simulink library "vmc"  (R2021b)
settings: Solver=VariableStepAuto  StartTime=0.0  StopTime=10.0  RelTol=1e-3
undefined symbols (not defined in the file): AVMC_ACCDeltaTqGradeGn_X_deg, AVMC_ACCDeltaTqIGain4OVRD_X_kph, AVMC_ACCDeltaTqIGain4OVRD_Y_mps2, AVMC_ACCDeltaTqIGain_X_kph, AVMC_ACCDeltaTqIGain_Y_mps2, AVMC_ACCDeltaTqPGain_X_kph, AVMC_ACCDeltaTqPGain_Y_kph, AVMC_ACCGradeofst_X_G, AVMC_ACCGradeofst_Y_pct, AVMC_ACCLoSpdTqLoLim4JP_X_kph, AVMC_ACCLoSpdTqLoLim4JP_Y_deg, AVMC_ACCLoSpdTqLowerLim_X_kph, AVMC_ACCLoSpdTqLowerLim_Y_deg, AVMC_ACCReqAccelGain_X_mps2, AVMC_ACCReqAccelGain_Y_enum, AVMC_ADSPosGFBDeltaTq_X_kph, AVMC_ADSPosGFBDeltaTq_Y_mps2, AVMC_AggressJerkPCT4AT_X_kph, AVMC_AggressJerkPCT_X_kph, AVMC_AggressLimitPCT4AT_X_kph, AVMC_AggressLimitPCT_X_kph, AVMC_DECGradeofst_X_G, AVMC_DECGradeofst_Y_pct, AVMC_DISCDeltaTqIGain_X_kph, AVMC_DISCDeltaTqIGain_Y_mps2, AVMC_DISCDeltaTqPGain_X_kph, AVMC_DISCDeltaTqPGain_Y_kph, AVMC_EPSForceSelect_X_enum, AVMC_EPSForceSelect_Y_enum, AVMC_EPSForceSelectD21_X_enum, AVMC_EPSForceSelectD21_Y_enum, AVMC_ESCRegenOut_X_kph, AVMC_ESCRegenOut_Y_Deg, AVMC_ESCRegenOutEnSpd_X_Deg, AVMC_EstPitchSlopeTs_X_kph, AVMC_GradeCompFlt_X_kph, AVMC_GyroYBandLo_X_Gps, AVMC_HoldResTq_X_kph, AVMC_ISOAccLimit_X_mps, AVMC_ISODecLimit_X_mps, AVMC_ISOJerk_X_mps, AVMC_LatESCRegenOut_X_kph, AVMC_LatESCRegenOut_Y_Deg, AVMC_LongAccDeadZone_X_kph, AVMC_LongAccFiltTsforP2_X_Gps, AVMC_MCPresBaseTq_X_bar, AVMC_MSAPedalOvrd_X_kph, AVMC_MSASpdBand_X_kph, AVMC_MSATqDownEndTq_X_kph, AVMC_MSATqDownTime_X_kph, AVMC_NegZCHoldTq_X_kph, AVMC_OPDDisSlideRate_X_Deg, AVMC_OVRD2ActSR2FCMCMD_X_mps2, AVMC_PedalTqRWhlRatio_X_Nm, AVMC_PedalTqRWhlRatio_Y_gps, AVMC_PedalTqRWhlSlipGain_X_rat, AVMC_PedalTqRWhlSlipGain_Y_kph, AVMC_PedalTqRWhSTRGGain_X_deg, AVMC_PedalTqRWhSTRGGain_Y_kph, AVMC_PosZCHoldTq_X_kph ... (+593)
libraries: hcu_lib x143, simulink x96, tqr x4, $bdroot x1, simulink_extras x1
(part 9 of 17)

== system vmc/VMC/VMC/ACC_Function/Hand Shaking ==
  VVMC_FeatArbitrFinal_enum : Inport
  VVMC_ACCCtrlAllow_flg : Inport  Port=2
  VVMC_ACCShutOffHold_flg : Inport  Port=3
  VINP_ADASACCSta_enum : Inport  Port=4
  VVMC_VMCACCCtrlAvail_flg : Inport  Port=5
  Constant1 : Constant  Value=TRUE
  Constant2 : Constant  Value=ENUM_FEATARBITRSTA_DISC
  Constant3 : Constant  Value=FALSE
  Constant4 : Constant  Value=ENUM_FEATARBITRSTA_ACC
  Constant5 : Constant  Value=TRUE
  Constant6 : Constant  Value=FALSE
  Constant7 : Constant  Value=ENUM_FEATARBITRSTA_AEB
  Constant9 : Constant  Value=ENUM_ADASACCSTA_ACTIVE
  Logical Operator : Logic  AllPortsSameDT=off  OutDataTypeStr=boolean
  Logical Operator1 : Logic  Operator=OR  Inputs=4  AllPortsSameDT=off  OutDataTypeStr=boolean
  Logical Operator2 : Logic  AllPortsSameDT=off  OutDataTypeStr=boolean
  OR1 : Logic  AllPortsSameDT=off  OutDataTypeStr=boolean
  Relational Operator{1..3,6} (4 alike) : RelationalOperator  Operator===  OutDataTypeStr=boolean  RndMeth=Simplest
  Switch : Switch  Criteria=u2 > Threshold
  u2>0 : Switch  Criteria=u2 > Threshold
  VVMC_ACCCtrlAvail_flg : Outport
  VVMC_ADASActive_flg : Outport  Port=2
  wires:
  VVMC_VMCACCCtrlAvail_flg/1 -> [VVMC_VMCACCCtrlAvail_flg]
  [VVMC_VMCACCCtrlAvail_flg] -> Logical Operator2/2
  [VVMC_ACCCtrlAllow_flg] -> Logical Operator2/1
  Relational Operator6/1 -> OR1/2
  Constant7/1 -> Relational Operator6/2
  [VVMC_FeatArbitrFinal_enum] -> Relational Operator6/1
  Relational Operator3/1 -> OR1/1
  VINP_ADASACCSta_enum/1 -> [VINP_ADASACCSta_enum]
  OR1/1 -> Logical Operator1/1
  Constant9/1 -> Relational Operator3/2
  [VINP_ADASACCSta_enum] -> Relational Operator3/1
  [VVMC_ACCShutOffHold_flg] -> Logical Operator1/2
  VVMC_ACCShutOffHold_flg/1 -> [VVMC_ACCShutOffHold_flg]
  Constant3/1 -> u2>0/3
  u2>0/1 -> [VVMC_ADASActive_flg]  "VVMC_ADASActive_flg"
  Constant1/1 -> u2>0/1
  Logical Operator/1 -> u2>0/2
  Relational Operator1/1 -> Logical Operator1/4
  VVMC_ACCCtrlAllow_flg/1 -> [VVMC_ACCCtrlAllow_flg]
  Constant5/1 -> Switch/1
  Constant6/1 -> Switch/3
  Switch/1 -> [VVMC_ACCCtrlAvail_flg]  "VVMC_ACCCtrlAvail_flg"
  Logical Operator2/1 -> Logical Operator/2, Switch/2
  [VVMC_ADASActive_flg] -> VVMC_ADASActive_flg/1
  Constant2/1 -> Relational Operator1/2
  [VVMC_FeatArbitrFinal_enum] -> Relational Operator1/1
  VVMC_FeatArbitrFinal_enum/1 -> [VVMC_FeatArbitrFinal_enum]
  [VVMC_ACCCtrlAvail_flg] -> VVMC_ACCCtrlAvail_flg/1
  [VVMC_FeatArbitrFinal_enum] -> Relational Operator2/1
  Constant4/1 -> Relational Operator2/2
  Relational Operator2/1 -> Logical Operator1/3
  Logical Operator1/1 -> Logical Operator/1

== system vmc/VMC/VMC/APS function/CAAS HandShake ==
  VVMC_VehicleSpeed_kph : Inport
  VVMC_ADASActive_flg : Inport  Port=2
  VVMC_CruzActive_flg : Inport  Port=3
  task_time_s : Inport  Port=4
  VINP_CAASVMCReqA_flg : Inport  Port=5
  AND : Logic  Inputs=3  AllPortsSameDT=off  OutDataTypeStr=boolean
  AND1 : Logic  AllPortsSameDT=off  OutDataTypeStr=boolean
  Constant1 : Constant  Value=KVMC_CAASCtrlAllowTime_s
  Constant11 : Constant  Value=KVMC_CAASEnVehSpd_kph
  Constant2 : Constant  Value=KVMC_CAASVMCReqA_flg_ovrdflg
  Constant3 : Constant  Value=KVMC_CAASVMCReqA_flg_ovrdval
  DelayEnable : hcu_lib/Basic_Blocks/DelayEnable
  NOT : Logic  Operator=NOT  AllPortsSameDT=off  OutDataTypeStr=boolean
  NOT1 : Logic  Operator=NOT  AllPortsSameDT=off  OutDataTypeStr=boolean
  Relational Operator : RelationalOperator  Operator=<=  OutDataTypeStr=boolean  RndMeth=Simplest
  Switch : Switch  Criteria=u2 > Threshold
  VVMC_CAASCtrlAvail_flg : Outport
  VVMC_CAASActive_flg : Outport  Port=2
  wires:
  Constant2/1 -> Switch/2
  Constant3/1 -> Switch/1
  Switch/1 -> AND1/2
  [VINP_CAASVMCReqA_flg] -> Switch/3
  [VVMC_CAASActive_flg] -> VVMC_CAASActive_flg/1
  AND1/1 -> [VVMC_CAASActive_flg]  "VVMC_CAASActive_flg"
  VINP_CAASVMCReqA_flg/1 -> [VINP_CAASVMCReqA_flg]
  [VVMC_CAASCtrlAvail_flg] -> AND1/1
  [VVMC_CAASCtrlAvail_flg] -> VVMC_CAASCtrlAvail_flg/1
  [VVMC_ADASActive_flg] -> NOT/1
  NOT/1 -> AND/2
  NOT1/1 -> AND/3
  [task_time_s] -> DelayEnable/3
  DelayEnable/1 -> [VVMC_CAASCtrlAvail_flg]  "VVMC_CAASCtrlAvail_flg"
  Constant11/1 -> Relational Operator/2
  VVMC_CruzActive_flg/1 -> [VVMC_CruzActive_flg]
  [VVMC_CruzActive_flg] -> NOT1/1
  [VVMC_VehicleSpeed_kph] -> Relational Operator/1
  task_time_s/1 -> [task_time_s]
  Constant1/1 -> DelayEnable/2
  AND/1 -> DelayEnable/1
  VVMC_VehicleSpeed_kph/1 -> [VVMC_VehicleSpeed_kph]
  VVMC_ADASActive_flg/1 -> [VVMC_ADASActive_flg]
  Relational Operator/1 -> AND/1

== system vmc/VMC/VMC/APS function/Command Determination1 ==
  VVMC_APSActive_flg : Inport
  VINP_APSStaSys_enum : Inport  Port=2
  VINP_APSShiftPosnReq_enum : Inport  Port=3
  VINP_APSSpeedCMD_kph : Inport  Port=4
  AND : Logic  AllPortsSameDT=off  OutDataTypeStr=boolean
  Constant : Constant  Value=ENUM_APSSYSTEMSTA_ACTIVE
  Constant1 : Constant  Value=ENUM_APSSYSTEMSTA_REMOTEACTIVE
  Constant2 : Constant  Value=ZERO_FLOAT
  Constant3 : Constant  Value=ENUM_APSSHIFTPOSNREQ_PARK
  Equal : RelationalOperator  Operator===  OutDataTypeStr=boolean  RndMeth=Simplest
  Equal1 : RelationalOperator  Operator===  OutDataTypeStr=boolean  RndMeth=Simplest
  OR : Logic  Operator=OR  AllPortsSameDT=off  OutDataTypeStr=boolean
  Switch : Switch  Criteria=u2 > Threshold
  Switch1 : Switch  Criteria=u2 > Threshold
  VVMC_APSSpeedCMD_kph : Outport
  VVMC_APSShiftPosnReq_enum : Outport  Port=2
  wires:
  VVMC_APSActive_flg/1 -> [VVMC_APSActive_flg]
  VINP_APSStaSys_enum/1 -> [VINP_APSStaSys_enum]
  VINP_APSShiftPosnReq_enum/1 -> [VINP_APSShiftPosnReq_enum]
  VINP_APSSpeedCMD_kph/1 -> [VINP_APSSpeedCMD_kph]
  [VINP_APSStaSys_enum] -> Equal/1
  Constant/1 -> Equal/2
  Constant1/1 -> Equal1/2
  [VINP_APSStaSys_enum] -> Equal1/1
  Equal/1 -> OR/1
  Equal1/1 -> OR/2
  [VVMC_APSActive_flg] -> AND/1
  OR/1 -> AND/2
  AND/1 -> [VVMC_APSEnCMD_flg]  "VVMC_APSEnCMD_flg"
  [VVMC_APSEnCMD_flg] -> Switch/2
  [VINP_APSSpeedCMD_kph] -> Switch/1
  Constant2/1 -> Switch/3
  Switch/1 -> VVMC_APSSpeedCMD_kph/1  "VVMC_APSSpeedCMD_kph"
  Switch1/1 -> VVMC_APSShiftPosnReq_enum/1  "VVMC_APSShiftPosnReq_enum"
  Constant3/1 -> Switch1/3
  [VINP_APSShiftPosnReq_enum] -> Switch1/1
  [VVMC_APSEnCMD_flg] -> Switch1/2

== system vmc/VMC/VMC/APS function/Hand Shake ==
  task_time_s : Inport
  VTQD_ExternalTqAllow_flg : Inport  Port=2
  VTQD_ExtShiftAllow_flg : Inport  Port=3
  VINP_APSVMCReqA_flg : Inport  Port=4
  VINP_APSStaSys_enum : Inport  Port=5
  VTQD_ExtDoorAllow_flg : Inport  Port=6
  VTQD_GearActualPosn_enum : Inport  Port=7
  VDDM_VCURAPSErrLv2_flg : Inport  Port=8
  VDDM_VCURAPSErrLv3_flg : Inport  Port=9
  VTQD_EPBCarWashMode_flg : Inport  Port=10
  AND : Logic  Inputs=4  AllPortsSameDT=off  OutDataTypeStr=boolean
  AND1 : Logic  Inputs=3  AllPortsSameDT=off  OutDataTypeStr=boolean
  AND2 : Logic  Inputs=4  AllPortsSameDT=off  OutDataTypeStr=boolean
  Constant : Constant  Value=KVMC_ExternalTqAllowTime_s
  Constant1 : Constant  Value=KVMC_ExternalShiftAllowTime_s
  Constant2 : Constant  Value=ENUM_APSSYSTEMSTA_ACTIVE
  Constant3 : Constant  Value=ENUM_APSSYSTEMSTA_REMOTEACTIVE
  Constant4 : Constant  Value=KVMC_ExternalDoorAllowTime_s
  Delay : Delay  DelayLength=1
  Delay1 : Delay  DelayLength=1
  DelayEnable : hcu_lib/Basic_Blocks/DelayEnable
  DelayEnable1 : hcu_lib/Basic_Blocks/DelayEnable
  DelayEnable2 : hcu_lib/Basic_Blocks/DelayEnable
  Detect Decrease : simulink/Logic and Bit Operations/Detect Decrease  vinit=0.0  OutDataTypeStr=boolean
  Equal : RelationalOperator  Operator===  OutDataTypeStr=boolean  RndMeth=Simplest
  Equal1 : RelationalOperator  Operator===  OutDataTypeStr=boolean  RndMeth=Simplest
  Logical Operator : Logic  Operator=NOT  AllPortsSameDT=off  OutDataTypeStr=boolean
  Logical Operator1 : Logic  Operator=NOT  AllPortsSameDT=off  OutDataTypeStr=boolean
  Logical Operator2 : Logic  Operator=NOT  AllPortsSameDT=off  OutDataTypeStr=boolean
  NOT : Logic  Operator=NOT  AllPortsSameDT=off  OutDataTypeStr=boolean
  OR : Logic  Operator=OR  AllPortsSameDT=off  OutDataTypeStr=boolean
  SR_Latch : hcu_lib/Basic_Blocks/SR_Latch
  Terminator : Terminator
  VVMC_APSCtrlAvail_flg : Outport
  VVMC_APSActive_flg : Outport  Port=2
  wires:
  [VVMC_APSActive_flg] -> Delay/1
  Delay/1 -> NOT/1
  Logical Operator1/1 -> AND/4
  Detect Decrease/1 -> SR_Latch/2
  Logical Operator2/1 -> AND/3
  [VVMC_APSActive_flg] -> Delay1/1
  [VDDM_VCURAPSErrLv2_flg] -> Logical Operator/1
  AND2/1 -> SR_Latch/1
  Delay1/1 -> Detect Decrease/1
  [VDDM_VCURAPSErrLv3_flg] -> Logical Operator2/1
  NOT/1 -> AND2/4
  [VTQD_EPBCarWashMode_flg] -> Logical Operator1/1
  [VVMC_APSShiftCtrlAllow_flg] -> AND2/1
  Logical Operator/1 -> AND2/3
  [VVMC_APSDoorCtrlAllow_flg] -> AND2/2
  SR_Latch/1 -> AND/2
  VTQD_EPBCarWashMode_flg/1 -> [VTQD_EPBCarWashMode_flg]
  VTQD_GearActualPosn_enum/1 -> [VTQD_GearActualPosn_enum]
  VDDM_VCURAPSErrLv2_flg/1 -> [VDDM_VCURAPSErrLv2_flg]
  VDDM_VCURAPSErrLv3_flg/1 -> [VDDM_VCURAPSErrLv3_flg]
  [VVMC_APSTqCtrlAllow_flg] -> AND/1
  AND/1 -> VVMC_APSCtrlAvail_flg/1, [VVMC_APSCtrlAvail_flg]  "VVMC_APSCtrlAvail_flg"
  [VTQD_ExtDoorAllow_flg] -> DelayEnable2/1
  [task_time_s] -> DelayEnable2/3
  DelayEnable2/1 -> [VVMC_APSDoorCtrlAllow_flg]  "VVMC_APSDoorCtrlAllow_flg"
  Constant4/1 -> DelayEnable2/2
  VTQD_ExtDoorAllow_flg/1 -> [VTQD_ExtDoorAllow_flg]
  VINP_APSStaSys_enum/1 -> [VINP_APSStaSys_enum]
  AND1/1 -> VVMC_APSActive_flg/1, [VVMC_APSActive_flg]  "VVMC_APSActive_flg"
  [VVMC_APSCtrlAvail_flg] -> AND1/2
  [VINP_APSStaSys_enum] -> Equal1/1
  Equal1/1 -> OR/2
  Constant3/1 -> Equal1/2
  [VINP_APSVMCReqA_flg] -> AND1/1
  OR/1 -> AND1/3
  Equal/1 -> OR/1
  [VINP_APSStaSys_enum] -> Equal/1
  Constant2/1 -> Equal/2
  [task_time_s] -> DelayEnable/3
  Constant/1 -> DelayEnable/2
  DelayEnable/1 -> [VVMC_APSTqCtrlAllow_flg]  "VVMC_APSTqCtrlAllow_flg"
  task_time_s/1 -> [task_time_s]
  VTQD_ExternalTqAllow_flg/1 -> [VTQD_ExternalTqAllow_flg]
  [VTQD_ExternalTqAllow_flg] -> DelayEnable/1
  [VTQD_ExtShiftAllow_flg] -> DelayEnable1/1
  DelayEnable1/1 -> [VVMC_APSShiftCtrlAllow_flg]  "VVMC_APSShiftCtrlAllow_flg"
  Constant1/1 -> DelayEnable1/2
  [task_time_s] -> DelayEnable1/3
  VTQD_ExtShiftAllow_flg/1 -> [VTQD_ExtShiftAllow_flg]
  VINP_APSVMCReqA_flg/1 -> [VINP_APSVMCReqA_flg]
  [VTQD_GearActualPosn_enum] -> Terminator/1

== system vmc/VMC/VMC/APS function/Signal Rounting ==
  VINP_SCPSystemMode_enum : Inport
  VVMC_APSActive_flg : Inport  Port=2
  VVMC_ADASActive_flg : Inport  Port=3
  VTQD_GearActualPosn_enum : Inport  Port=4
  VVMC_CAASActive_flg : Inport  Port=5
  VTQD_APSStaSys_enum : Inport  Port=6
  VTQD_APSDecReqA_flg : Inport  Port=7
  VTQD_APSDecReq_mps2 : Inport  Port=8
  VTQD_APSReq_enum : Inport  Port=9
  VINP_APSStaSystem_enum : Inport  Port=10
  VINP_APSDecReqA_flg : Inport  Port=11
  VINP_APSDecReq_mps2 : Inport  Port=12
  VINP_APSReq_enum : Inport  Port=13
  VVMC_SetACCDisableAPS_flg : Inport  Port=14
  Signal Determination VINP_APSDecReqAtest_flg : Subsystem
  Signal Determination VINP_APSDecReqtest_mps2 : Subsystem
  Signal Determination VINP_APSReqtest_enum : Subsystem
  Signal Determination VINP_APSStaSystemtest_enum : Subsystem
  Switch{,1..3} (4 alike) : Switch  Criteria=u2 > Threshold
  VVMC_APSStaSys_enum : Outport
  VVMC_APSDecReqA_flg : Outport  Port=2
  VVMC_APSDecReq_mps2 : Outport  Port=3
  VVMC_APSReq_enum : Outport  Port=4
  wires:
  [VINP_APSReq_enum] -> Switch3/1
  [VTQD_APSReq_enum] -> Switch3/3
  [VVMC_SetACCDisableAPS_flg] -> Switch3/2
  [VINP_APSDecReq_mps2] -> Switch2/1
  [VTQD_APSDecReq_mps2] -> Switch2/3
  [VVMC_SetACCDisableAPS_flg] -> Switch2/2
  [VINP_APSDecReqA_flg] -> Switch1/1
  [VTQD_APSDecReqA_flg] -> Switch1/3
  [VVMC_SetACCDisableAPS_flg] -> Switch1/2
  [VTQD_APSStaSys_enum] -> Switch/3
  [VINP_APSStaSystem_enum] -> Switch/1
  [VVMC_SetACCDisableAPS_flg] -> Switch/2
  VVMC_SetACCDisableAPS_flg/1 -> [VVMC_SetACCDisableAPS_flg]
  [VINP_APSStaSystem_enum] -> Signal Determination VINP_APSStaSystemtest_enum/1(SignalInput1)
  [VINP_APSDecReqA_flg] -> Signal Determination VINP_APSDecReqAtest_flg/1(SignalInput1)
  [VINP_APSDecReq_mps2] -> Signal Determination VINP_APSDecReqtest_mps2/1(SignalInput1)
  VINP_APSDecReq_mps2/1 -> [VINP_APSDecReq_mps2]
  VINP_APSReq_enum/1 -> [VINP_APSReq_enum]
  VINP_APSDecReqA_flg/1 -> [VINP_APSDecReqA_flg]
  VINP_APSStaSystem_enum/1 -> [VINP_APSStaSystem_enum]
  Switch3/1 -> Signal Determination VINP_APSReqtest_enum/2(SignalInput2)
  Switch2/1 -> Signal Determination VINP_APSDecReqtest_mps2/2(SignalInput2)
  Switch1/1 -> Signal Determination VINP_APSDecReqAtest_flg/2(SignalInput2)
  Switch/1 -> Signal Determination VINP_APSStaSystemtest_enum/2(SignalInput2)
  VTQD_APSStaSys_enum/1 -> [VTQD_APSStaSys_enum]
  VTQD_APSDecReqA_flg/1 -> [VTQD_APSDecReqA_flg]
  VTQD_APSReq_enum/1 -> [VTQD_APSReq_enum]
  VTQD_APSDecReq_mps2/1 -> [VTQD_APSDecReq_mps2]
  [VVMC_CAASActive_flg] -> Signal Determination VINP_APSReqtest_enum/6(VVMC_CAASActive_flg)
  [VVMC_CAASActive_flg] -> Signal Determination VINP_APSDecReqtest_mps2/6(VVMC_CAASActive_flg)
  [VVMC_CAASActive_flg] -> Signal Determination VINP_APSDecReqAtest_flg/6(VVMC_CAASActive_flg)
  [VVMC_CAASActive_flg] -> Signal Determination VINP_APSStaSystemtest_enum/7(VVMC_CAASActive_flg)
  VVMC_CAASActive_flg/1 -> [VVMC_CAASActive_flg]
  [VINP_APSReq_enum] -> Signal Determination VINP_APSReqtest_enum/1(SignalInput1)
  [VINP_SCPSystemMode_enum] -> Signal Determination VINP_APSStaSystemtest_enum/3(VINP_SCPSystemMode_enum)
  [VTQD_GearActualPosn_enum] -> Signal Determination VINP_APSStaSystemtest_enum/6(VTQD_GearActualPosn_enum)
  VTQD_GearActualPosn_enum/1 -> [VTQD_GearActualPosn_enum]
  [VVMC_ADASActive_flg] -> Signal Determination VINP_APSReqtest_enum/5(VVMC_ADASActive_flg)
  [VVMC_APSActive_flg] -> Signal Determination VINP_APSReqtest_enum/4(VVMC_APSActive_flg)
  [VVMC_ADASActive_flg] -> Signal Determination VINP_APSDecReqtest_mps2/5(VVMC_ADASActive_flg)
  [VVMC_APSActive_flg] -> Signal Determination VINP_APSDecReqtest_mps2/4(VVMC_APSActive_flg)
  [VVMC_ADASActive_flg] -> Signal Determination VINP_APSDecReqAtest_flg/5(VVMC_ADASActive_flg)
  [VVMC_APSActive_flg] -> Signal Determination VINP_APSDecReqAtest_flg/4(VVMC_APSActive_flg)
  [VVMC_ADASActive_flg] -> Signal Determination VINP_APSStaSystemtest_enum/5(VVMC_ADASActive_flg)
  [VVMC_APSActive_flg] -> Signal Determination VINP_APSStaSystemtest_enum/4(VVMC_APSActive_flg)
  VVMC_ADASActive_flg/1 -> [VVMC_ADASActive_flg]
  VVMC_APSActive_flg/1 -> [VVMC_APSActive_flg]
  VINP_SCPSystemMode_enum/1 -> [VINP_SCPSystemMode_enum]
  Signal Determination VINP_APSDecReqtest_mps2/1(SignalOutp) -> VVMC_APSDecReq_mps2/1  "VVMC_APSDecReq_mps2"
  [VINP_SCPSystemMode_enum] -> Signal Determination VINP_APSDecReqAtest_flg/3(VINP_SCPSystemMode_enum)
  Signal Determination VINP_APSStaSystemtest_enum/1(SignalOutp) -> VVMC_APSStaSys_enum/1  "VVMC_APSStaSys_enum"
  [VINP_SCPSystemMode_enum] -> Signal Determination VINP_APSReqtest_enum/3(VINP_SCPSystemMode_enum)
  Signal Determination VINP_APSReqtest_enum/1(SignalOutp) -> VVMC_APSReq_enum/1  "VVMC_APSReq_enum"
  Signal Determination VINP_APSDecReqAtest_flg/1(SignalOutp) -> VVMC_APSDecReqA_flg/1  "VVMC_APSDecReqA_flg"
  [VINP_SCPSystemMode_enum] -> Signal Determination VINP_APSDecReqtest_mps2/3(VINP_SCPSystemMode_enum)

== system vmc/VMC/VMC/APS function/Subsystem ==
  VINP_ADASACCSta_enum : Inport
  VINP_MCPressure_bar : Inport  Port=2
  VINP_BrkSwSta_flg : Inport  Port=3
  VINP_BrkPedalPos_pct : Inport  Port=4
  VTQD_APSDecReqA_flg : Inport  Port=5
  VINP_ACCObjDist_m : Inport  Port=6
  VVMC_MeterIndSpeedForCalcu_kph : Inport  Port=7
  VVMC_VehicleSpeed_kph : Inport  Port=8
  0 : Constant  Value=KVMC_AllowSetSpdOvrd_flg
  1 : Constant  Value=KVMC_AllowSetSpdOvrdVal_flg
  2m : Constant  Value=KVMC_NotAllowSetSpdDist_m
  6m : Constant  Value=KVMC_AllowSetSpdDist_m
  AND : Logic  Inputs=6  AllPortsSameDT=off  OutDataTypeStr=boolean
  AND1 : Logic  Operator=OR  AllPortsSameDT=off  OutDataTypeStr=boolean
  AND3 : Logic  AllPortsSameDT=off  OutDataTypeStr=boolean
  Constant1 : Constant  Value=ENUM_ADASACCSTA_ACTIVE
  Constant2 : Constant  Value=ENUM_ADASACCSTA_STANDBY
  Constant4 : Constant  Value=KVMC_APSAllowSetACCMCP_bar
  Constant5 : Constant  Value=ZERO_FLOAT
  Constant6 : Constant  Value=TRUE
  Constant7 : Constant  Value=KVMC_APSAllowSetACCPosn_pct
  NOT : Logic  Operator=NOT  AllPortsSameDT=off  OutDataTypeStr=boolean
  NOT1 : Logic  Operator=NOT  AllPortsSameDT=off  OutDataTypeStr=boolean
  Relational Operator : RelationalOperator  Operator===  OutDataTypeStr=boolean  RndMeth=Simplest
  Relational Operator1 : RelationalOperator  Operator===  OutDataTypeStr=boolean  RndMeth=Simplest
  Relational Operator{2..4,6} (4 alike) : RelationalOperator  Operator=>  OutDataTypeStr=boolean  RndMeth=Simplest
  Relational Operator5 : RelationalOperator  Operator=<=  OutDataTypeStr=boolean  RndMeth=Simplest
  SR_Latch2 : hcu_lib/Basic_Blocks/SR_Latch
  Switch : Switch  Criteria=u2 > Threshold
  Switch1 : Switch  Criteria=u2 > Threshold
  Terminator : Terminator
  VVMC_SetACCDisableAPS_flg : Outport
  wires:
  VVMC_VehicleSpeed_kph/1 -> [VVMC_VehicleSpeed_kph]
  [VTQD_APSDecReqA_flg] -> Switch/2
  VTQD_APSDecReqA_flg/1 -> [VTQD_APSDecReqA_flg]
  [VINP_BrkSwSta_flg] -> AND/3
  VINP_BrkPedalPos_pct/1 -> [VINP_BrkPedalPos_pct]
  VINP_MCPressure_bar/1 -> [VINP_MCPressure_bar]
  VINP_ADASACCSta_enum/1 -> [VINP_ADASACCSta_enum]
  VVMC_MeterIndSpeedForCalcu_kph/1 -> [VVMC_MeterIndSpeedForCalcu_kph]
  VINP_ACCObjDist_m/1 -> [VINP_ACCObjDist_m]
  AND3/1 -> Switch1/3
  Switch1/1 -> [VVMC_AllowSetSpd_flg]  "VVMC_AllowSetSpd_flg"
  0/1 -> Switch1/2
  Relational Operator5/1 -> AND3/1
  2m/1 -> Relational Operator6/2
  [VINP_ACCObjDist_m] -> Relational Operator5/1, Relational Operator6/1
  1/1 -> Switch1/1
  Relational Operator6/1 -> AND3/2
  6m/1 -> Relational Operator5/2
  Relational Operator2/1 -> AND/4
  SR_Latch2/1 -> Switch/1
  [VINP_ADASACCSta_enum] -> Relational Operator/1
  [VINP_ADASACCSta_enum] -> Relational Operator1/1
  Constant1/1 -> Relational Operator1/2
  [VINP_BrkPedalPos_pct] -> Relational Operator4/1
  Constant4/1 -> Relational Operator2/2
  Constant7/1 -> Relational Operator4/2
  NOT/1 -> AND1/2
  VINP_BrkSwSta_flg/1 -> [VINP_BrkSwSta_flg]
  [VINP_BrkSwSta_flg] -> NOT/1
  [VVMC_AllowSetSpd_flg] -> AND/2
  [VINP_MCPressure_bar] -> Relational Operator2/1
  [VVMC_VehicleSpeed_kph] -> Relational Operator3/1
  Switch/1 -> VVMC_SetACCDisableAPS_flg/1  "VVMC_SetACCDisableAPS_flg"
  AND1/1 -> SR_Latch2/2
  Relational Operator/1 -> AND/1
  Constant5/1 -> Relational Operator3/2
  Relational Operator3/1 -> NOT1/1
  Constant2/1 -> Relational Operator/2
  Relational Operator1/1 -> AND1/1
  AND/1 -> SR_Latch2/1
  Relational Operator4/1 -> AND/5
  Constant6/1 -> Switch/3
  NOT1/1 -> AND/6
  [VVMC_MeterIndSpeedForCalcu_kph] -> Terminator/1

== system vmc/VMC/VMC/CruiseControlFunction/CCActiveDetermination ==
  VTQD_SpdCtrlMode_enum : Inport
  VVMC_FeatArbitrFinal_enum : Inport  Port=2
  VTQD_ExternalTqAllow_flg : Inport  Port=3
  VTQD_SWC1SetdownSta_flg : Inport  Port=4
  VTQD_SWC1ResUpSta_flg : Inport  Port=5
  VVMC_VehicleSpeed_kph : Inport  Port=6
  VVMC_FeatSetSpdFinal_raw32 : Inport  Port=7
  VINP_BrakeSWGPIO_flg : Inport  Port=8
  VTQD_SWC1CANCELSta_flg : Inport  Port=9
  VINP_BrkSwSta_flg : Inport  Port=10
  VINP_ADASAEBSta_enum : Inport  Port=11
  VVMC_CCPedalOvrd_flg : Inport  Port=12
  VTQD_GearActualPosn_enum : Inport  Port=13
  VINP_Distanceunit_flg : Inport  Port=14
  VTQD_ExtDoorAllow_flg : Inport  Port=15
  VVMC_VMCCCCtrlAvail_flg : Inport  Port=16
  VVMC_MeterIndSpeed_raw32 : Inport  Port=17
  " 1" : Constant  Value=KTQD_CCActiveMetSpdLo_kph
  " 2" : Constant  Value=KTQD_CCActiveMetSpdLoMPH_mph
  1 : Constant  Value=KPH2MPH
  3 : Constant  Value=KTQD_CCActiveMetSpdHi_kph
  5 : Constant  Value=KTQD_CCActiveMetSpdHiMPH_mph
  AND : Logic  AllPortsSameDT=off  OutDataTypeStr=boolean
  Cast To Single : DataTypeConversion  OutDataTypeStr=uint8
  Cast To Single1 : DataTypeConversion  OutDataTypeStr=boolean
  Cast To Single2 : DataTypeConversion  OutDataTypeStr=boolean
  Cast To Single3 : DataTypeConversion  OutDataTypeStr=single
  Cast To Single4 : DataTypeConversion  OutDataTypeStr=single
  Chart : Stateflow chart  TreatAsAtomicUnit=on
      settings: PortSchema="{\"entries\":[{\"content\":{\"sides\":[{\"content\":{\"connectorIds\":[\"In1\",\"In2\",\"In3\",\"In4\",\"In19\",\"In5\",\"In6\",\"In7\",\"In8\",\"In9\",\"In10\",\"In11\",\"In12\",\"In13\",\"In14\",\"In15\",\"In16\",\"In17\",\"In18\"]},\"type\":\"ConnectorPlacement.EquallySpacedRectSide\",\"uuid\":\"729a9221-d173-4bb4-827a-23a519ff93ff\"},{\"content\":{\"connectorIds\":[\"Out1\",\"Out2\"],\"side\":\"RIGHT\"},\"type\":\"ConnectorPlacement.EquallySpacedRectSide\",\"uuid\":\"6a4c923b-ece4-4666-bd9b-e2812ecb47ad\"},{\"content\":{\"connectorIds\":[],\"side\":\"TOP\"},\"type\":\"ConnectorPlacement.EquallySpacedRectSide\",\"uuid\":\"86a2c43e-d83c-4805-8909-bdaa1b82f756\"}]},\"type\":\"ConnectorPlacement.EquallySpacedConnector\",\"uuid\":\"7c9222a8-b3d3-4fae-b3b9-9a17496e8fb9\"}],\"packageUris\":[\"http://schema.mathworks.com/mf0/Connector/R2020b\"],\"version\":\"1.0\"}"
  Constant2 : Constant  Value=KVMC_CCMSASpdWar_kph
  Constant3 : Constant  Value=ENUM_FEATARBITRSTA_CC
  Constant4 : Constant  Value=TRUE
  Constant5 : Constant  Value=FALSE
  Constant6 : Constant  Value=ENUM_CCCRLSTA_ACTIVE
  Constant7 : Constant  Value=ENUM_ADASAEBSTA_ACTIVE
  Constant8 : Constant  Value=ENUM_GEARACTUALPOSN_D
  Delay : Delay  DelayLength=1
  Detect Decrease : simulink/Logic and Bit Operations/Detect Decrease  vinit=0.0  OutDataTypeStr=boolean
  Detect Decrease1 : simulink/Logic and Bit Operations/Detect Decrease  vinit=0.0  OutDataTypeStr=boolean
  Detect Decrease2 : simulink/Logic and Bit Operations/Detect Decrease  vinit=0.0  OutDataTypeStr=boolean
  Divide : Product  Inputs=**
  Relational Operator : RelationalOperator  Operator===  OutDataTypeStr=boolean  RndMeth=Simplest
  Relational Operator1 : RelationalOperator  Operator===  OutDataTypeStr=boolean  RndMeth=Simplest
  Switch1 : Switch  Criteria=u2 > Threshold
  Switch2 : Switch  Criteria=u2 > Threshold
  Switch3 : Switch  Criteria=u2 > Threshold
  Terminator : Terminator
  u2 > 0 : Switch  Criteria=u2 > Threshold
  VVMC_CCCtrlSta_enum : Outport
  VVMC_CCSpdWar_flg : Outport  Port=2
  VVMC_CruzActive_flg : Outport  Port=3
  wires:
  [VVMC_VMCCCCtrlAvail_flg] -> Chart/18(VVMC_VMCCCCtrlAvail_flg)
  VVMC_VMCCCCtrlAvail_flg/1 -> [VVMC_VMCCCCtrlAvail_flg]
  [VTQD_ExtDoorAllow_flg] -> Chart/17(VTQD_ExtDoorAllow_flg)
  VTQD_ExtDoorAllow_flg/1 -> [VTQD_ExtDoorAllow_flg]
  Cast To Single4/1 -> Chart/5(KVMC_CCActiveMetSpdLo_kph)
  Cast To Single3/1 -> Chart/4(KVMC_CCActiveMetSpdHi_kph)
  VINP_Distanceunit_flg/1 -> [VINP_Distanceunit_flg]
  " 1"/1 -> Switch3/3
  [VINP_Distanceunit_flg] -> Switch3/2
  " 2"/1 -> Switch3/1
  [VINP_Distanceunit_flg] -> Switch2/2
  5/1 -> Switch2/1
  3/1 -> Switch2/3
  Constant8/1 -> Chart/16(ENUM_GEARACTUALPOSN_D)
  [VTQD_GearActualPosn_enum] -> Chart/15(VTQD_GearActualPosn_enum)
  VTQD_GearActualPosn_enum/1 -> [VTQD_GearActualPosn_enum]
  [VINP_BrkSwSta_flg] -> Chart/10(VINP_BrkSwSta_flg)
  Cast To Single/1 -> [VVMC_CCCtrlSta_enum]  "VVMC_CCCtrlSta_enum"
  Cast To Single2/1 -> [VVMC_CruzActive_flg]  "VVMC_CruzActive_flg"
  Cast To Single1/1 -> [VVMC_CCSpdWar_flg]  "VVMC_CCSpdWar_flg"
  Detect Decrease2/1 -> Chart/11(VVMC_DetectSWCResUp_flg)  "VVMC_DetectSWCResUp_flg"
  Detect Decrease1/1 -> Chart/9(VVMC_DetectSWCCANCEL_flg)  "VVMC_DetectSWCCANCEL_flg"
  Detect Decrease/1 -> Chart/3(VVMC_DetectSWCSetDown_flg)  "VVMC_DetectSWCSetDown_flg"
  [VVMC_CruzActive_flg] -> VVMC_CruzActive_flg/1
  [VVMC_CCSpdWar_flg] -> VVMC_CCSpdWar_flg/1
  [VVMC_CCCtrlSta_enum] -> VVMC_CCCtrlSta_enum/1
  VINP_BrkSwSta_flg/1 -> [VINP_BrkSwSta_flg]
  VTQD_SWC1CANCELSta_flg/1 -> [VTQD_SWC1CANCELSta_flg]
  VINP_BrakeSWGPIO_flg/1 -> [VINP_BrakeSWGPIO_flg]
  VVMC_FeatSetSpdFinal_raw32/1 -> [VVMC_FeatSetSpdFinal_raw32]
  VVMC_VehicleSpeed_kph/1 -> [VVMC_VehicleSpeed_kph]
  VTQD_SWC1ResUpSta_flg/1 -> [VTQD_SWC1ResUpSta_flg]
  VTQD_SWC1SetdownSta_flg/1 -> [VTQD_SWC1SetdownSta_flg]
  VTQD_ExternalTqAllow_flg/1 -> [VTQD_ExternalTqAllow_flg]
  VVMC_FeatArbitrFinal_enum/1 -> [VVMC_FeatArbitrFinal_enum]
  u2 > 0/1 -> Cast To Single2/1
  Chart/2(VVMC_CCSpdWar_flg) -> Cast To Single1/1
  Chart/1(VVMC_CCCtrlSta_enum) -> Cast To Single/1
  [VTQD_SWC1ResUpSta_flg] -> Detect Decrease2/1
  [VTQD_SWC1CANCELSta_flg] -> Detect Decrease1/1
  [VINP_BrakeSWGPIO_flg] -> Chart/8(VINP_BrakeSWGPIO_flg)
  [VVMC_FeatArbitrFinal_enum] -> Relational Operator/1
  [VTQD_ExternalTqAllow_flg] -> Chart/2(VTQD_ExternalTqAllow_flg)
  Switch1/1 -> Chart/7(KVMC_CCMSASpdWar_raw32)
  [VVMC_FeatSetSpdFinal_raw32] -> Chart/6(VVMC_FeatSetSpdFinal_raw32)
  [VTQD_SWC1SetdownSta_flg] -> Detect Decrease/1
  Switch3/1 -> Cast To Single4/1
  Switch2/1 -> Cast To Single3/1
  Constant3/1 -> Relational Operator/2
  VTQD_SpdCtrlMode_enum/1 -> [VTQD_SpdCtrlMode_enum]
  [VTQD_SpdCtrlMode_enum] -> Chart/1(VTQD_SpdCtrlMode_enum)
  AND/1 -> u2 > 0/2
  Constant4/1 -> u2 > 0/1
  Constant5/1 -> u2 > 0/3
  Constant6/1 -> Relational Operator1/2
  [VVMC_CCCtrlSta_enum] -> Relational Operator1/1
  Relational Operator/1 -> AND/1
  Relational Operator1/1 -> AND/2
  VINP_ADASAEBSta_enum/1 -> [VINP_ADASAEBSta_enum]
  [VINP_ADASAEBSta_enum] -> Chart/12(VINP_ADASAEBSta_enum)
  Constant7/1 -> Chart/13(ENUM_ADASAEBSTA_ACTIVE)
  VVMC_CCPedalOvrd_flg/1 -> [VVMC_CCPedalOvrd_flg]
  [VVMC_CCPedalOvrd_flg] -> Delay/1
  Delay/1 -> Chart/14(VVMC_CCPedalOvrd_flg)
  [VVMC_MeterIndSpeed_raw32] -> Chart/19(VVMC_MeterIndSpeed_raw32)
  1/1 -> Divide/1
  Constant2/1 -> Switch1/3, Divide/2
  [VINP_Distanceunit_flg] -> Switch1/2
  Divide/1 -> Switch1/1
  VVMC_MeterIndSpeed_raw32/1 -> [VVMC_MeterIndSpeed_raw32]
  [VVMC_VehicleSpeed_kph] -> Terminator/1

== system vmc/VMC/VMC/CruiseControlFunction/CCDemandTorqueCalculation ==
  VVMC_FeatSetSpdForCalcu_kph : Inport
  VVMC_VehicleSpeed_kph : Inport  Port=2
  VVMC_CruzActive_flg : Inport  Port=3
  VVMC_LongAcc_Gps : Inport  Port=4
  VVMC_CCPedalOvrd_flg : Inport  Port=5
  VVMC_ActACCRequiredAccel_mps2 : Inport  Port=6
  VVMC_SafetyCtrl_flg : Inport  Port=7
  VTQR_FrTMTqReq_Nm : Inport  Port=8
  VTQR_RrTMTqReq_Nm : Inport  Port=9
  VVMC_TotalAvailBrkRgnTq_Nm : Inport  Port=10
  VINP_RDCActive_enum : Inport  Port=11
  AND1 : Logic  AllPortsSameDT=off  OutDataTypeStr=boolean
  AND12 : Logic  AllPortsSameDT=off  OutDataTypeStr=boolean
  Abs3 : Abs
  Abs4 : Abs
  Add{8,12,16,20..21} (5 alike) : Sum
  Add22 : Sum  Inputs=+-
  Add23 : Sum  Inputs=+-
  Cast To Single4 : DataTypeConversion  OutDataTypeStr=single
  Cast To Single5 : DataTypeConversion  OutDataTypeStr=single
  Constant1 : Constant  Value=KVMC_CCTqUpLim_Nm
  Constant104 : Constant  Value=ZERO_FLOAT
  Constant105 : Constant  Value=KTQD_RrTMTotalGearRatio_gain
  Constant106 : Constant  Value=KTQR_RrTMGearEff_c
  Constant107 : Constant  Value=KVMC_GravityValue_mps2
  Constant145 : Constant  Value=ENUM_CANRDCACTSTA_EXITIMMEDIATELY
  Constant2 : Constant  Value=KVMC_CCTqLowLim_Nm
  Constant3 : Constant  Value=ZERO_FLOAT
  Constant36 : Constant  Value=KVMC_AccDevLowLim_mps2
  Constant38 : Constant  Value=KVMC_AccDevUpLim_mps2
  Constant4 : Constant  Value=KVMC_CCDISCPGainSW_flg
  Constant40 : Constant  Value=KVMC_CCSpdDevUpLim_kph
  Constant5 : Constant  Value=KVMC_CCTqUpLim_Nm
  Constant56 : Constant  Value=KVMC_CCSpdDevLowLim_kph
  Constant58 : Constant  Value=KVMC_Veh2MeterSpdFactor_enum
  Constant59 : Constant  Value=KVMC_Veh2MeterSpdOffset_enum
  Constant6 : Constant  Value=KVMC_CCTqLowLim_Nm
  Constant64 : Constant  Value=KVMC_TqSafetyCtrl_flg
  Constant65 : Constant  Value=KVMC_Veh2MeterSpdLoFactor_enum
  Constant7 : Constant  Value=ZERO_FLOAT
  Constant71 : Constant  Value=KTQR_FrTMGearEff_c
  Constant76 : Constant  Value=KTQD_FrTMTotalGearRatio_gain
  Data Type Conversion1 : DataTypeConversion  OutDataTypeStr=single
  Detect Decrease3 : simulink/Logic and Bit Operations/Detect Decrease  vinit=0.0  OutDataTypeStr=boolean
  Detect Increase3 : simulink/Logic and Bit Operations/Detect Increase  vinit=0.0  OutDataTypeStr=boolean
  Divide11 : Product  Inputs=**
  Divide12 : Product  Inputs=**
  Divide4 : Product  Inputs=***
  Divide7 : Product  Inputs=***
  InitialCondition: 1 : UnitDelay  SampleTime=-1  HasFrameUpgradeWarning=on
  Logical Operator1 : Logic  Operator=OR  AllPortsSameDT=off  OutDataTypeStr=boolean
  MVMC_DISCDeltaTqIGain_Z_Nm : Lookup_n-D  BreakpointsForDimension1=AVMC_DISCDeltaTqIGain_Y_mps2  BreakpointsForDimension2=AVMC_DISCDeltaTqIGain_X_kph  Table=MVMC_DISCDeltaTqIGain_Z_Nm  InternalRulePriority=Speed  RndMeth=Simplest  InputSameDT=on
      settings: InputPortMap=u0,u1
  MVMC_DISCDeltaTqPGain_Z_Nm : Lookup_n-D  BreakpointsForDimension1=AVMC_DISCDeltaTqPGain_Y_kph  BreakpointsForDimension2=AVMC_DISCDeltaTqPGain_X_kph  BreakpointsForDimension3=[5, 7]  Table=MVMC_DISCDeltaTqPGain_Z_Nm  ExtrapMethod=Clip  InternalRulePriority=Speed  RndMeth=Simplest  InputSameDT=on
      settings: InputPortMap=u0,u1
  Max : MinMax  Function=max  Inputs=2
  Max1 : MinMax  Function=max  Inputs=2
  Product2 : Product
  Relational Operator1 : RelationalOperator  Operator=~=  OutDataTypeStr=boolean  RndMeth=Simplest
  Relational Operator18 : RelationalOperator  Operator=<=  OutDataTypeStr=boolean  RndMeth=Simplest
  Saturation Dynamic{1,7..9} (4 alike) : simulink/Discontinuities/Saturation Dynamic  OutMin=[]  OutMax=[]  OutDataTypeStr=Inherit: Same as second input  OutDataType=fixdt(1, 16)  OutScaling=2^-10  DoSatur=off
  Switch{,2,5,7} (4 alike) : Switch  Criteria=u2 > Threshold
  Switch1 : Switch  Criteria=u2 > Threshold  Threshold=KVMC_Veh2MeterSpdLoBdy_kph
  Unit Delay3 : UnitDelay  SampleTime=-1  HasFrameUpgradeWarning=on
  u2 > 0 (3)1 : Switch  Criteria=u2 > Threshold
  u2 > 0 (4)1 : Switch  Criteria=u2 > Threshold
  VVMC_CruzWhlTqCal_Nm : Outport
  wires:
  Constant3/1 -> Switch/3
  MVMC_DISCDeltaTqPGain_Z_Nm/1 -> Switch/1
  [VVMC_CruzActive_flg] -> Switch/2
  Add21/1 -> Saturation Dynamic1/2
  Constant1/1 -> Saturation Dynamic1/1
  Constant2/1 -> Max1/1
  [VVMC_TotalAvailBrkRgnTq_Nm] -> Max1/2
  Max1/1 -> Saturation Dynamic1/3
  Divide12/1 -> Switch1/3
  Divide11/1 -> Add8/2
  Constant65/1 -> Divide12/2
  Constant58/1 -> Divide11/1
  Add8/1 -> Switch1/1
  Constant59/1 -> Add8/1
  Switch1/1 -> Add23/2
  [VVMC_VehicleSpeed_kph] -> Divide12/1, Switch1/2, Divide11/2
  Saturation Dynamic1/1 -> [VVMC_CruzWhlTqCal_Nm]  "VVMC_CruzWhlTqCal_Nm"
  Constant7/1 -> Switch2/3
  Constant4/1 -> Switch2/2
  [VVMC_CCPGainDeltaTq_Nm] -> Switch2/1
  Switch2/1 -> Add21/1
  Switch/1 -> [VVMC_CCPGainDeltaTq_Nm]  "VVMC_CCPGainDeltaTq_Nm"
  Max/1 -> Saturation Dynamic7/3
  [VVMC_TotalAvailBrkRgnTq_Nm] -> Max/2
  VVMC_TotalAvailBrkRgnTq_Nm/1 -> [VVMC_TotalAvailBrkRgnTq_Nm]
  VTQR_RrTMTqReq_Nm/1 -> [VTQR_RrTMTqReq_Nm]
  VTQR_FrTMTqReq_Nm/1 -> [VTQR_FrTMTqReq_Nm]
  Cast To Single4/1 -> u2 > 0 (3)1/3, Abs4/1, u2 > 0 (4)1/3
  Constant56/1 -> Saturation Dynamic9/3
  Constant6/1 -> Max/1
  Constant36/1 -> Saturation Dynamic8/3
  [VVMC_LongAcc_Gps] -> Product2/1
  Product2/1 -> Add22/2
  Constant38/1 -> Saturation Dynamic8/1
  Logical Operator1/1 -> Switch7/2
  [VVMC_FeatSetSpdForCalcu_kph] -> Data Type Conversion1/1
  Constant64/1 -> AND12/1
  Constant107/1 -> Product2/2
  Add22/1 -> Saturation Dynamic8/2
  [VVMC_CCReqAcc_mps2] -> Add22/1
  Unit Delay3/1 -> Detect Decrease3/1
  Add16/1 -> Add20/1
  Constant5/1 -> Saturation Dynamic7/1
  Constant40/1 -> Saturation Dynamic9/1
  Add12/1 -> Switch7/3
  Switch7/1 -> Cast To Single4/1
  Cast To Single5/1 -> Saturation Dynamic7/2
  [VVMC_CCPedalOvrd_flg] -> Unit Delay3/1
  [VVMC_CruzActive_flg] -> AND1/1
  Constant105/1 -> Divide7/2
  Add20/1 -> Switch7/1
  AND12/1 -> u2 > 0 (3)1/2
  Divide7/1 -> Add16/2
  Constant76/1 -> Divide4/2
  [VVMC_CCIGainDeltaTq_Nm] -> Add20/2
  Saturation Dynamic8/1 -> MVMC_DISCDeltaTqIGain_Z_Nm/1
  [VTQR_FrTMTqReq_Nm] -> Divide4/1
  Abs3/1 -> Relational Operator18/1
  Saturation Dynamic7/1 -> Add21/2, InitialCondition: 1/1
  Abs4/1 -> Relational Operator18/2
  [VVMC_CCIGainDeltaTq_Nm] -> Add12/2
  [VVMC_VehicleSpeed_kph] -> MVMC_DISCDeltaTqIGain_Z_Nm/2
  Detect Increase3/1 -> Logical Operator1/1
  InitialCondition: 1/1 -> [VVMC_LastCCWhlTqCalW_Nm]  "VVMC_LastCruzWhlTqCal_Nm"
  Constant104/1 -> Switch5/3
  Add23/1 -> Saturation Dynamic9/2
  MVMC_DISCDeltaTqIGain_Z_Nm/1 -> [VVMC_CCIGainDeltaTq_Nm]  "VVMC_CCIGainDeltaTq_Nm"
  [VVMC_LastCCWhlTqCalW_Nm] -> Add12/1
  [VTQR_RrTMTqReq_Nm] -> Divide7/1
  u2 > 0 (4)1/1 -> u2 > 0 (3)1/1  "VVMC_CruzWhlTqCalAftSafety_Nm"
  [VVMC_LastCCWhlTqCalW_Nm] -> u2 > 0 (4)1/1, Abs3/1
  Relational Operator18/1 -> u2 > 0 (4)1/2
  Saturation Dynamic9/1 -> MVMC_DISCDeltaTqPGain_Z_Nm/1
  [VVMC_SafetyCtrl_flg] -> AND12/2
  Constant106/1 -> Divide7/3
  Constant71/1 -> Divide4/3
  u2 > 0 (3)1/1 -> Switch5/1
  Data Type Conversion1/1 -> Add23/1
  [VVMC_FeatSetSpdForCalcu_kph] -> MVMC_DISCDeltaTqPGain_Z_Nm/2
  [VVMC_CruzActive_flg] -> Detect Increase3/1
  Divide4/1 -> Add16/1
  Detect Decrease3/1 -> Logical Operator1/2
  Switch5/1 -> Cast To Single5/1
  VVMC_SafetyCtrl_flg/1 -> [VVMC_SafetyCtrl_flg]
  VVMC_ActACCRequiredAccel_mps2/1 -> [VVMC_CCReqAcc_mps2]
  VVMC_CCPedalOvrd_flg/1 -> [VVMC_CCPedalOvrd_flg]
  VVMC_LongAcc_Gps/1 -> [VVMC_LongAcc_Gps]
  [VVMC_CruzWhlTqCal_Nm] -> VVMC_CruzWhlTqCal_Nm/1
  VVMC_VehicleSpeed_kph/1 -> [VVMC_VehicleSpeed_kph]
  VVMC_CruzActive_flg/1 -> [VVMC_CruzActive_flg]
  VVMC_FeatSetSpdForCalcu_kph/1 -> [VVMC_FeatSetSpdForCalcu_kph]
  [VINP_RDCActive_enum] -> Relational Operator1/1
  Constant145/1 -> Relational Operator1/2
  Relational Operator1/1 -> AND1/2
  AND1/1 -> Switch5/2
  VINP_RDCActive_enum/1 -> [VINP_RDCActive_enum]

== system vmc/VMC/VMC/CruiseControlFunction/CCTorqueSourceDetermination ==
  VTQD_DriverWhlTqDem_Nm : Inport
  VVMC_CruzWhlTqCal_Nm : Inport  Port=2
  VTQD_LowIdleAccPedal_flg : Inport  Port=3
  VTQD_RegenMode_enum : Inport  Port=4
  VVMC_FeatArbitrFinal_enum : Inport  Port=5
  task_time_s : Inport  Port=6
  AND1 : Logic  Inputs=3  AllPortsSameDT=off  OutDataTypeStr=boolean
  Add : Sum
  Constant20 : Constant  Value=FALSE
  Constant21 : Constant  Value=ENUM_FEATARBITRSTA_CC
  Constant22 : Constant  Value=TRUE
  Constant23 : Constant  Value=KVMC_ACCPedalOvrdRestTime_s
  DelayEnable : hcu_lib/Basic_Blocks/DelayEnable
  Direct Lookup Table (n-D)1 : LookupNDDirect  NumberOfTableDimensions=1  Table=MVMC_ACCPedalOvrdTqHys_Y_Nm
  NOT2 : Logic  Operator=NOT  AllPortsSameDT=off  OutDataTypeStr=boolean
  OR1 : Logic  Operator=OR  AllPortsSameDT=off  OutDataTypeStr=boolean
  Relational Operator6 : RelationalOperator  Operator===  OutDataTypeStr=boolean  RndMeth=Simplest
  Relational Operator7 : RelationalOperator  Operator=>  OutDataTypeStr=boolean  RndMeth=Simplest
  Relational Operator8 : RelationalOperator  Operator=<=  OutDataTypeStr=boolean  RndMeth=Simplest
  SR_Latch : hcu_lib/Basic_Blocks/SR_Latch
  u2 > 0 (1) : Switch  Criteria=u2 > Threshold
  u2 > 0 (2) : Switch  Criteria=u2 > Threshold
  VVMC_CruzWhlTqReq_Nm : Outport
  VVMC_CCPedalOvrd_flg : Outport  Port=2
  wires:
  task_time_s/1 -> [task_time_s]
  VVMC_FeatArbitrFinal_enum/1 -> [VVMC_FeatArbitrFinal_enum]
  VTQD_RegenMode_enum/1 -> [VTQD_RegenMode_enum]
  Constant22/1 -> u2 > 0 (2)/1
  Direct Lookup Table (n-D)1/1 -> Add/2
  Constant21/1 -> Relational Operator6/2
  AND1/1 -> u2 > 0 (2)/2, u2 > 0 (1)/2
  [VTQD_LowIdleAccPedal_flg] -> OR1/2
  SR_Latch/1 -> [VVMC_CCPedalTqEnOvrd_flg]  "VVMC_CCPedalTqEnOvrd_flg"
  DelayEnable/1 -> OR1/1
  [VTQD_DriverWhlTqDem_Nm] -> Relational Operator8/1
  [VTQD_RegenMode_enum] -> Direct Lookup Table (n-D)1/1
  Relational Operator6/1 -> AND1/1
  Constant20/1 -> u2 > 0 (2)/3
  NOT2/1 -> AND1/2
  [VVMC_CCPedalTqEnOvrd_flg] -> AND1/3
  Relational Operator7/1 -> SR_Latch/1
  u2 > 0 (1)/1 -> [VVMC_CruzWhlTqReq_Nm]
  Constant23/1 -> DelayEnable/2
  Relational Operator8/1 -> DelayEnable/1
  OR1/1 -> SR_Latch/2
  [VVMC_FeatArbitrFinal_enum] -> Relational Operator6/1
  [VTQD_DriverWhlTqDem_Nm] -> Relational Operator7/1
  Add/1 -> Relational Operator7/2
  u2 > 0 (2)/1 -> [VVMC_CCPedalOvrd_flg]
  [VVMC_CruzWhlTqCal_Nm] -> Add/1
  [VVMC_CruzWhlTqCal_Nm] -> Relational Operator8/2
  [VVMC_CruzWhlTqCal_Nm] -> u2 > 0 (1)/3
  [VTQD_DriverWhlTqDem_Nm] -> u2 > 0 (1)/1
  [VTQD_LowIdleAccPedal_flg] -> NOT2/1
  [task_time_s] -> DelayEnable/3
  [VVMC_CCPedalOvrd_flg] -> VVMC_CCPedalOvrd_flg/1
  VTQD_LowIdleAccPedal_flg/1 -> [VTQD_LowIdleAccPedal_flg]
  [VVMC_CruzWhlTqReq_Nm] -> VVMC_CruzWhlTqReq_Nm/1
  VVMC_CruzWhlTqCal_Nm/1 -> [VVMC_CruzWhlTqCal_Nm]
  VTQD_DriverWhlTqDem_Nm/1 -> [VTQD_DriverWhlTqDem_Nm]

== system vmc/VMC/VMC/IMU/IMU memorized offset result ==
  VINP_MemOffsetGyroX_raw16 : Inport
  VINP_MemOffsetGyroY_raw16 : Inport  Port=2
  VINP_MemOffsetGyroZ_raw16 : Inport  Port=3
  VINP_MemOffsetAccX_raw16 : Inport  Port=4
  VINP_MemOffsetAccY_raw16 : Inport  Port=5
  VINP_MemOffsetAccZ_raw16 : Inport  Port=6
  ACCEL_FS_SEL = 001 SENSITIVITY = 2000 LSB/g : Constant  Value=KVMC_AccFSCalSet_enum
  Constant6 : Constant  Value=ONE_FLOAT  OutDataTypeStr=single
  Data Type Conversion : DataTypeConversion  OutDataTypeStr=uint16
  Data Type Conversion{1..6} (6 alike) : DataTypeConversion  OutDataTypeStr=single
  Data Type Conversion7 : DataTypeConversion  OutDataTypeStr=uint16
  Divide{,1..5} (6 alike) : Product  Inputs=**
  GYRO_FS_SEL = 0001 SENSITIVITY = 50 LSB/dps : Constant  Value=KVMC_GyroFSCalSet_enum
  Math Function{,1..5} (6 alike) : Math  Operator=reciprocal  SaturateOnIntegerOverflow=on
  Plus : Sum  Inputs=+-
  VVMC_MemOffsetGyroX_Dps : Outport
  VVMC_MemOffsetGyroY_Dps : Outport  Port=2
  VVMC_MemOffsetGyroZ_Dps : Outport  Port=3
  VVMC_MemOffsetAccX_G : Outport  Port=4
  VVMC_MemOffsetAccY_G : Outport  Port=5
  VVMC_MemOffsetAccZ_G : Outport  Port=6
  wires:
  Data Type Conversion6/1 -> Math Function5/1
  Data Type Conversion5/1 -> Math Function4/1
  Data Type Conversion4/1 -> Math Function3/1
  Data Type Conversion3/1 -> Math Function2/1
  Data Type Conversion2/1 -> Math Function1/1
  Data Type Conversion1/1 -> Math Function/1
  Math Function5/1 -> Divide5/2
  Math Function4/1 -> Divide4/2
  Math Function3/1 -> Divide3/2
  Math Function2/1 -> Divide2/2
  Math Function1/1 -> Divide1/2
  Math Function/1 -> Divide/2
  VINP_MemOffsetAccZ_raw16/1 -> [VINP_MemOffsetAccZ_raw16]
  VINP_MemOffsetAccY_raw16/1 -> [VINP_MemOffsetAccY_raw16]
  VINP_MemOffsetAccX_raw16/1 -> [VINP_MemOffsetAccX_raw16]
  VINP_MemOffsetGyroZ_raw16/1 -> [VINP_MemOffsetGyroZ_raw16]
  Divide4/1 -> [VVMC_MemOffsetAccY_G]  "VVMC_MemOffsetAccY_G"
  [VVMC_MemOffsetAccZ_G] -> VVMC_MemOffsetAccZ_G/1
  [VVMC_MemOffsetAccY_G] -> VVMC_MemOffsetAccY_G/1
  [VVMC_MemOffsetAccX_G] -> VVMC_MemOffsetAccX_G/1
  [VVMC_MemOffsetGyroZ_Dps] -> VVMC_MemOffsetGyroZ_Dps/1
  [VVMC_MemOffsetGyroY_Dps] -> VVMC_MemOffsetGyroY_Dps/1
  [VVMC_MemOffsetGyroX_Dps] -> VVMC_MemOffsetGyroX_Dps/1
  Constant6/1 -> Plus/2
  Divide5/1 -> Plus/1
  Plus/1 -> [VVMC_MemOffsetAccZ_G]  "VVMC_MemOffsetAccZ_G"
  Divide3/1 -> [VVMC_MemOffsetAccX_G]  "VVMC_MemOffsetAccX_G"
  Divide2/1 -> [VVMC_MemOffsetGyroZ_Dps]  "VVMC_MemOffsetGyroZ_Dps"
  Divide1/1 -> [VVMC_MemOffsetGyroY_Dps]  "VVMC_MemOffsetGyroY_Dps"
  Divide/1 -> [VVMC_MemOffsetGyroX_Dps]  "VVMC_MemOffsetGyroX_Dps"
  ACCEL_FS_SEL = 001 SENSITIVITY = 2000 LSB/g/1 -> Data Type Conversion7/1
  Data Type Conversion7/1 -> [VVMC_AccFSCalSet_enum]  "VVMC_AccFSCalSet_enum"
  [VINP_MemOffsetAccZ_raw16] -> Divide5/1
  [VVMC_AccFSCalSet_enum] -> Data Type Conversion6/1
  [VVMC_AccFSCalSet_enum] -> Data Type Conversion5/1
  [VINP_MemOffsetAccY_raw16] -> Divide4/1
  [VINP_MemOffsetAccX_raw16] -> Divide3/1
  [VVMC_AccFSCalSet_enum] -> Data Type Conversion4/1
  [VVMC_GyroFSCalSet_enum] -> Data Type Conversion3/1
  [VINP_MemOffsetGyroZ_raw16] -> Divide2/1
  [VINP_MemOffsetGyroY_raw16] -> Divide1/1
  [VVMC_GyroFSCalSet_enum] -> Data Type Conversion2/1
  Data Type Conversion/1 -> [VVMC_GyroFSCalSet_enum]  "VVMC_GyroFSCalSet_enum"
  GYRO_FS_SEL = 0001 SENSITIVITY = 50 LSB/dps/1 -> Data Type Conversion/1
  [VVMC_GyroFSCalSet_enum] -> Data Type Conversion1/1
  [VINP_MemOffsetGyroX_raw16] -> Divide/1
  VINP_MemOffsetGyroY_raw16/1 -> [VINP_MemOffsetGyroY_raw16]
  VINP_MemOffsetGyroX_raw16/1 -> [VINP_MemOffsetGyroX_raw16]
